simulink model "Aircraft6dof"  (R2023b)
settings: Solver=ode4  StartTime=startTime  StopTime=stopTime  FixedStep=stepTime  RelTol=1e-3  EnableMultiTasking=on
values from neighbouring files (symbols this model uses):
  a0_s2 = 0    [SetupForTrimAndLin_Aircraft6dof.m]
  a0_s3 = 0    [SetupForTrimAndLin_Aircraft6dof.m]
  a0_s4 = 0.05    [SetupForTrimAndLin_Aircraft6dof.m]
  a0_s5 = 0.05    [SetupForTrimAndLin_Aircraft6dof.m]
  AR_s2 = b_s2 / c_s2    [SetupForTrimAndLin_Aircraft6dof.m]
  AR_s3 = b_s3 / c_s3    [SetupForTrimAndLin_Aircraft6dof.m]
  AR_s4 = (b_s4+b_s5) / c_s4    [SetupForTrimAndLin_Aircraft6dof.m]
  AR_s5 = (b_s4+b_s5) / c_s5    [SetupForTrimAndLin_Aircraft6dof.m]
  ARvecP1 = ARvecUIUCp1 * 30/pi * 2    [SetupForTrimAndLin_Aircraft6dof.m]
  c_s2 = componentMassesAndGeom(3,2)    [SetupForTrimAndLin_Aircraft6dof.m]
  c_s3 = componentMassesAndGeom(4,2)    [SetupForTrimAndLin_Aircraft6dof.m]
  c_s4 = componentMassesAndGeom(1,2)    [SetupForTrimAndLin_Aircraft6dof.m]
  c_s5 = componentMassesAndGeom(2,2)    [SetupForTrimAndLin_Aircraft6dof.m]
  CD0_s2 = 0.01    [SetupForTrimAndLin_Aircraft6dof.m]
  CD0_s3 = 0.01    [SetupForTrimAndLin_Aircraft6dof.m]
  CD0_s4 = 0.01    [SetupForTrimAndLin_Aircraft6dof.m]
  CD0_s5 = 0.01    [SetupForTrimAndLin_Aircraft6dof.m]
  CDa_s2 = 1    [SetupForTrimAndLin_Aircraft6dof.m]
  CDa_s3 = 1    [SetupForTrimAndLin_Aircraft6dof.m]
  CDa_s4 = 1    [SetupForTrimAndLin_Aircraft6dof.m]
  CDa_s5 = 1    [SetupForTrimAndLin_Aircraft6dof.m]
  CL0_s2 = 0    [SetupForTrimAndLin_Aircraft6dof.m]
  CL0_s3 = 0    [SetupForTrimAndLin_Aircraft6dof.m]
  CL0_s4 = 0.05    [SetupForTrimAndLin_Aircraft6dof.m]
  CL0_s5 = 0.05    [SetupForTrimAndLin_Aircraft6dof.m]
  CM0_s2 = 0    [SetupForTrimAndLin_Aircraft6dof.m]
  CM0_s3 = 0    [SetupForTrimAndLin_Aircraft6dof.m]
  CM0_s4 = -0.05    [SetupForTrimAndLin_Aircraft6dof.m]
  CM0_s5 = -0.05    [SetupForTrimAndLin_Aircraft6dof.m]
  CMa_s2 = 0    [SetupForTrimAndLin_Aircraft6dof.m]
  CMa_s3 = 0    [SetupForTrimAndLin_Aircraft6dof.m]
  CMa_s4 = 0    [SetupForTrimAndLin_Aircraft6dof.m]
  CMa_s5 = 0    [SetupForTrimAndLin_Aircraft6dof.m]
  CQvecP1 = CPvecP1    [SetupForTrimAndLin_Aircraft6dof.m]
  CTvecP1 = CTvecUIUCp1 * 2 * (1/(2*pi))^2 * (2^4)    [SetupForTrimAndLin_Aircraft6dof.m]
  dCL_du = 3    [SetupForTrimAndLin_Aircraft6dof.m]
  dE_0 = 0    [SetupForTrimAndLin_Aircraft6dof.m]
  dEL_0 = 0    [SetupForTrimAndLin_Aircraft6dof.m]
  DeMixMatrix = inv(MixMatrix)    [SetupForTrimAndLin_Aircraft6dof.m]
  dER_0 = 0    [SetupForTrimAndLin_Aircraft6dof.m]
  dR_0 = 0    [SetupForTrimAndLin_Aircraft6dof.m]
  e_s2 = 0.8    [SetupForTrimAndLin_Aircraft6dof.m]
  e_s3 = 0.8    [SetupForTrimAndLin_Aircraft6dof.m]
  e_s4 = 0.9    [SetupForTrimAndLin_Aircraft6dof.m]
  e_s5 = 0.9    [SetupForTrimAndLin_Aircraft6dof.m]
  elevator_vector = [0  0  0.1    0.1   -0.1    -0.1  0       0  ]    [SetupAndRun_Aircraft6dof.m]
  g_E_N = [0; 0; 9.81]*1    [SetupAndRun_Aircraft6dof.m]    (also in SetupForTrimAndLin_Aircraft6dof.m = [0; 0; 9.81])
  i_s2 = -0.1    [SetupForTrimAndLin_Aircraft6dof.m]
  i_s3 = 0    [SetupForTrimAndLin_Aircraft6dof.m]
  i_s4 = 0.0    (= 0)    [SetupForTrimAndLin_Aircraft6dof.m]
  i_s5 = 0.0    (= 0)    [SetupForTrimAndLin_Aircraft6dof.m]
  InitAtt = InitAtt_deg * deg2rad    [SetupAndRun_Aircraft6dof.m]    (also in SetupForTrimAndLin_Aircraft6dof.m)
  InitPos = InitPos_deg .* [deg2rad; deg2rad; 1]    [SetupAndRun_Aircraft6dof.m]    (also in SetupForTrimAndLin_Aircraft6dof.m)
  InitRates = Rates_Trim    [SetupAndRun_Aircraft6dof.m]    (also in SetupForTrimAndLin_Aircraft6dof.m = [0; 0; 0])
  InitVel = Vel_B_BA_Trim    [SetupAndRun_Aircraft6dof.m]    (also in SetupForTrimAndLin_Aircraft6dof.m = [15; 0; 0])
  Io_motor = 1.6    [SetupForTrimAndLin_Aircraft6dof.m]
  J = zeros(3,3)    [DefineAircraftGeometry.m]    (also in InitializeModel.m = ASW.RotationalInertiaMatrix; SetupAndRun_Aircraft6dof.m = [0.049 0 -0.0004; 0 0.022 0; -0.0004 0 0.071]; SetupForTrimAndLin_Aircraft6dof.m)
  Ki_motor = 0.009549    [SetupForTrimAndLin_Aircraft6dof.m]
  m = sum(obj.componentMassesAndGeom(:,1))    [DefineAircraftGeometry.m]    (also in SetupForTrimAndLin_Aircraft6dof.m = sum(componentMassesAndGeom(:,1)))
  MixMatrix = [-1 1 0 0 ... (first row only)    [SetupForTrimAndLin_Aircraft6dof.m]
  n_p1 = [1; 0; 0]    [SetupForTrimAndLin_Aircraft6dof.m]
  n_s2 = [0; 0; -1]    [SetupForTrimAndLin_Aircraft6dof.m]
  n_s3 = [0; 1; 0]    [SetupForTrimAndLin_Aircraft6dof.m]
  n_s4 = [0; sin(0*pi/180);  -cos(0*pi/180)]    [SetupForTrimAndLin_Aircraft6dof.m]
  n_s5 = [0; sin(0*pi/180);  -cos(0*pi/180)]    [SetupForTrimAndLin_Aircraft6dof.m]
  nCellsSeries = 6    [SetupForTrimAndLin_Aircraft6dof.m]
  om_motor_init = 0    [SetupForTrimAndLin_Aircraft6dof.m]
  R_p1 = componentMassesAndGeom(11,3)/2    [SetupForTrimAndLin_Aircraft6dof.m]
  Rearth = 6371000    [SetupForTrimAndLin_Aircraft6dof.m]
  Rmotor = 0.4    [SetupForTrimAndLin_Aircraft6dof.m]
  rudder_vector = [0  0  -0.1   -0.1 0      0     0.1     0.1   0       0  ]    [SetupAndRun_Aircraft6dof.m]
  S_s2 = c_s2 * b_s2    [SetupForTrimAndLin_Aircraft6dof.m]
  S_s3 = c_s3 * b_s3    [SetupForTrimAndLin_Aircraft6dof.m]
  S_s4 = c_s4 * b_s4    [SetupForTrimAndLin_Aircraft6dof.m]
  S_s5 = c_s5 * b_s5    [SetupForTrimAndLin_Aircraft6dof.m]
  S_u_s2 = c_u_s2*b_s2    [SetupForTrimAndLin_Aircraft6dof.m]
  S_u_s3 = c_u_s3*b_s3    [SetupForTrimAndLin_Aircraft6dof.m]
  S_u_s4 = c_u_s4*b_s4    [SetupForTrimAndLin_Aircraft6dof.m]
  S_u_s5 = c_u_s5*b_s5    [SetupForTrimAndLin_Aircraft6dof.m]
  tauE = 0.1    [SetupForTrimAndLin_Aircraft6dof.m]
  tauEL = 0.1    [SetupForTrimAndLin_Aircraft6dof.m]
  tauER = 0.1    [SetupForTrimAndLin_Aircraft6dof.m]
  tauR = 0.1    [SetupForTrimAndLin_Aircraft6dof.m]
  time_vector_elevator = [0  10 10.001 100   100.001 200   200.001 10000]    [SetupAndRun_Aircraft6dof.m]
  time_vector_rudder = [0  10 10.001 70   70.001 200   200.001 300   300.001 10000]    [SetupAndRun_Aircraft6dof.m]
  v_N_AE = [0; 0; 0]    [SetupAndRun_Aircraft6dof.m]    (also in SetupForTrimAndLin_Aircraft6dof.m)
  VcellMax = 4.2    [SetupForTrimAndLin_Aircraft6dof.m]
  Vel_W_Trim = [norm(Vel_B_BA_Trim); atan2(Vel_B_BA_Trim(3),Vel_B_BA_Trim(1)); asin(Vel_B_BA_Trim(2)/norm(Vel_B_BA_Trim)) ]    [TrimAndLinearize_ATT_wInputs_Aircraft6dof.m]
  x_cm = sum(obj.componentMassesAndGeom(:,1) .* obj.componentMassesAndGeom(:,5:7)) / m    [DefineAircraftGeometry.m]    (also in SetupForTrimAndLin_Aircraft6dof.m = x_cm')
  x_p1 = componentMassesAndGeom(11,5:7)'    [SetupForTrimAndLin_Aircraft6dof.m]
  x_s2 = [componentMassesAndGeom(3,5) + (1/4)*componentMassesAndGeom(3,2); componentMassesAndGeom(3,6);componentMassesAndGeom(3,7)]    [SetupForTrimAndLin_Aircraft6dof.m]
  x_s3 = [componentMassesAndGeom(4,5) + (1/4)*componentMassesAndGeom(4,2); componentMassesAndGeom(4,6);componentMassesAndGeom(4,7)]    [SetupForTrimAndLin_Aircraft6dof.m]
  x_s4 = [componentMassesAndGeom(1,5) + (1/4)*componentMassesAndGeom(1,2); componentMassesAndGeom(1,6);componentMassesAndGeom(1,7)]    [SetupForTrimAndLin_Aircraft6dof.m]
  x_s5 = [componentMassesAndGeom(2,5) + (1/4)*componentMassesAndGeom(2,2); componentMassesAndGeom(2,6);componentMassesAndGeom(2,7)]    [SetupForTrimAndLin_Aircraft6dof.m]
undefined symbols (not defined in the file or in its folder): InitQuat, J_int, K_decouple, K_lqr, n_int, reg_lqg, X_trim, Y_trim
libraries: vrlib x8, simulink x7, aerolibfltsims x1
(part 3 of 3)

== matlab function Aircraft6dof/Actuators - Plant - Sensors/Compute Wind Axes Vector/Compute Wind DCMs ==
  data: Vinf input; C_SB output; C_WB output; alpha input; beta input
function [C_SB, C_WB] = fcn(Vinf, alpha, beta)
%#codegen

C_SB = [cos(alpha)   0   sin(alpha) ;
        0           1   0         ;
        -sin(alpha)  0   cos(alpha)];
    
C_WS = [cos(beta)   sin(beta)   0 ;
        -sin(beta)  cos(beta)   0 ;
        0           0           1];
C_WB = C_WS * C_SB;

== matlab function Aircraft6dof/Actuators - Plant - Sensors/Equations Of Motion State Equations/Rot Kin (Orientation) Euler/MATLAB Function ==
  data: ATT input; MATRIX output
function MATRIX = EulerIntegrationMatrix(ATT)
%#codegen

phi=ATT(1);
theta=ATT(2);
psi=ATT(3);

MATRIX = [1     sin(phi)*tan(theta)   cos(phi)*tan(theta) ; 
          0     cos(phi)             -sin(phi)            ;
          0     sin(phi)/cos(theta)   cos(phi)/cos(theta)   ];

== matlab function Aircraft6dof/Actuators - Plant - Sensors/Equations Of Motion State Equations/MATLAB Function ==
  data: ATT input; DCM output
function DCM = ATT2DCM(ATT)
%#codegen

phi=ATT(1);
theta=ATT(2);
psi=ATT(3);

DCM = [ cos(theta)*cos(psi)                             cos(theta)*sin(psi)                            -sin(theta)          ; 
        sin(theta)*cos(psi)*sin(phi)-sin(psi)*cos(phi)  sin(theta)*sin(psi)*sin(phi)+cos(psi)*cos(phi)  cos(theta)*sin(phi) ;
        sin(theta)*cos(psi)*cos(phi)+sin(psi)*sin(phi)  sin(theta)*sin(psi)*cos(phi)-cos(psi)*sin(phi)  cos(theta)*cos(phi)   ];
